simulink model "FinalProjesi"  (R2025b)
settings: Solver=VariableStepAuto  StartTime=0.0  StopTime=10.0  RelTol=1e-3
libraries: simulink_extras x4
settings Model: Creator=ahmet  LastModifiedBy=ahmet

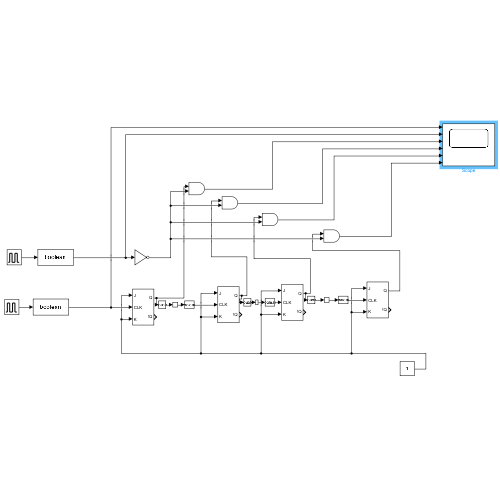
[thumbnail: Simulink's stored preview of the top-level diagram]
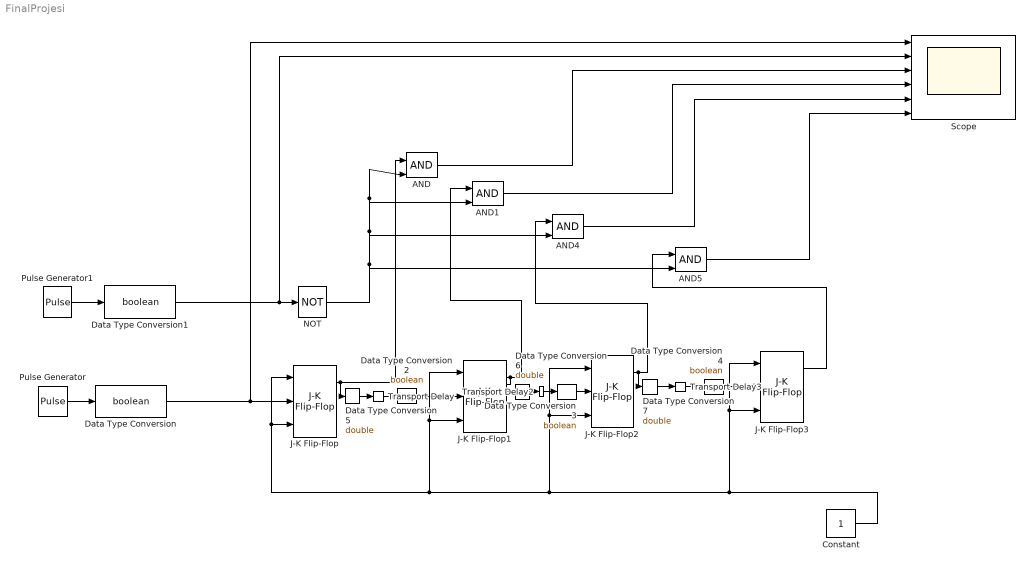
== system FinalProjesi ==
  AND{,1,4..5} (4 alike) : Logic  IconShape=distinctive  AllPortsSameDT=off  OutDataTypeStr=boolean
  Constant : Constant  OutDataTypeStr=boolean
  Data Type Conversion{,1..4} (5 alike) : DataTypeConversion  OutDataTypeStr=boolean  SaturateOnIntegerOverflow=off  RndMeth=Floor
  Data Type Conversion5 : DataTypeConversion  OutDataTypeStr=double  SaturateOnIntegerOverflow=off  RndMeth=Floor
  Data Type Conversion6 : DataTypeConversion  OutDataTypeStr=double  SaturateOnIntegerOverflow=off  RndMeth=Floor
  Data Type Conversion7 : DataTypeConversion  OutDataTypeStr=double  SaturateOnIntegerOverflow=off  RndMeth=Floor
  J-K Flip-Flop{,1..3} (4 alike) : simulink_extras/Flip Flops/J-K Flip-Flop  initial_condition=0
  NOT : Logic  Operator=NOT  IconShape=distinctive  AllPortsSameDT=off  OutDataTypeStr=boolean
  Pulse Generator : DiscretePulseGenerator  PulseType=Time based  Period=1  PulseWidth=50
  Pulse Generator1 : DiscretePulseGenerator  PulseType=Time based  Period=100  PulseWidth=5
  Scope : Scope  NumInputPorts=6
      settings: ActiveDisplayYMinimum=-0.12499999999999997  ActiveDisplayYMaximum=1.125
  Transport Delay : TransportDelay  DelayTime=150e-12
  Transport Delay2 : TransportDelay  DelayTime=150e-12
  Transport Delay3 : TransportDelay  DelayTime=150e-12
  wires:
  J-K Flip-Flop1/1 -> Data Type Conversion6/1, AND1/1
  J-K Flip-Flop2/1 -> AND4/1, Data Type Conversion7/1
  Constant/1 -> J-K Flip-Flop1/3, J-K Flip-Flop1/1, J-K Flip-Flop/3, J-K Flip-Flop/1, J-K Flip-Flop2/3, J-K Flip-Flop2/1, J-K Flip-Flop3/3, J-K Flip-Flop3/1
  NOT/1 -> AND5/2, AND4/2, AND1/2, AND/2
  J-K Flip-Flop3/1 -> AND5/1
  Pulse Generator/1 -> Data Type Conversion/1
  Data Type Conversion/1 -> J-K Flip-Flop/2, Scope/1
  Pulse Generator1/1 -> Data Type Conversion1/1
  Data Type Conversion1/1 -> Scope/2, NOT/1
  J-K Flip-Flop/1 -> Data Type Conversion5/1, AND/1
  Transport Delay/1 -> Data Type Conversion2/1
  Data Type Conversion2/1 -> J-K Flip-Flop1/2
  Data Type Conversion3/1 -> J-K Flip-Flop2/2
  Transport Delay2/1 -> Data Type Conversion3/1
  Transport Delay3/1 -> Data Type Conversion4/1
  Data Type Conversion4/1 -> J-K Flip-Flop3/2
  Data Type Conversion5/1 -> Transport Delay/1
  Data Type Conversion6/1 -> Transport Delay2/1
  Data Type Conversion7/1 -> Transport Delay3/1
  AND/1 -> Scope/3
  AND1/1 -> Scope/4
  AND4/1 -> Scope/5
  AND5/1 -> Scope/6
